simulink model "2"  (R2019a)
settings: Solver=VariableStepAuto  StartTime=0.0  StopTime=10.0  RelTol=1e-3
settings Model: Creator=TakumiShiota  LastModifiedBy=TakumiShiota

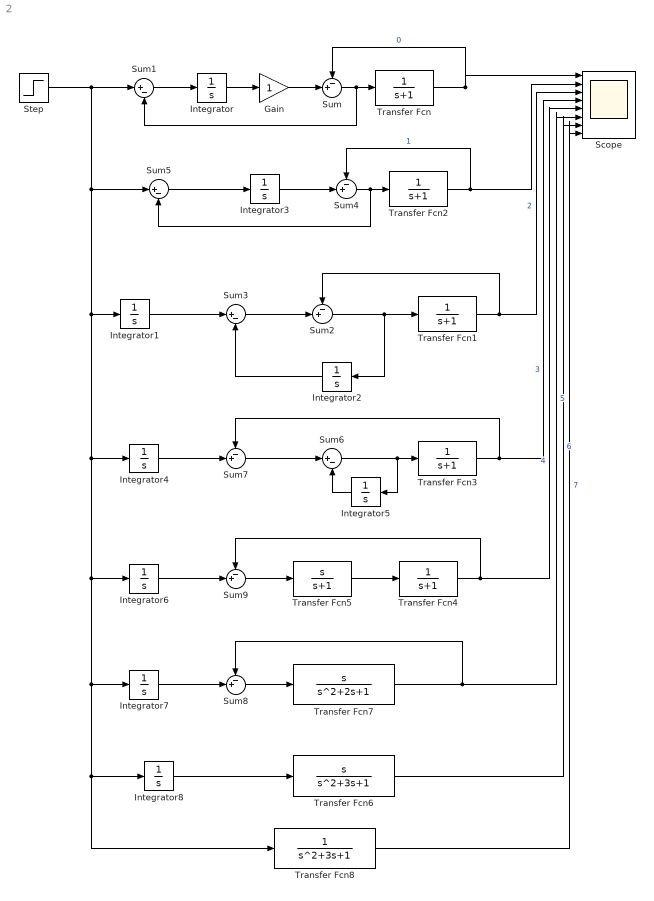
== system 2 ==
  Gain : Gain
  Integrator{,1..8} (9 alike) : Integrator
  Scope : Scope  NumInputPorts=8
  Step : Step  SampleTime=0
  Sum{,2,4,7..9} (6 alike) : Sum  Inputs=-+|
  Sum{1,3,5..6} (4 alike) : Sum  Inputs=|+-
  Transfer Fcn{,1..4} (5 alike) : TransferFcn  Denominator=[1 1]
  Transfer Fcn5 : TransferFcn  Numerator=[1 0]  Denominator=[1 1]
  Transfer Fcn6 : TransferFcn  Numerator=[1 0]  Denominator=[1 3 1]
  Transfer Fcn7 : TransferFcn  Numerator=[1 0]
  Transfer Fcn8 : TransferFcn  Denominator=[1 3 1]
  wires:
  Integrator/1 -> Gain/1
  Gain/1 -> Sum/2
  Sum/1 -> Sum1/2, Transfer Fcn/1
  Transfer Fcn/1 -> Sum/1, Scope/1  "0"
  Sum1/1 -> Integrator/1
  Sum3/1 -> Sum2/2
  Sum2/1 -> Integrator2/1, Transfer Fcn1/1
  Integrator2/1 -> Sum3/2
  Integrator1/1 -> Sum3/1
  Transfer Fcn1/1 -> Sum2/1, Scope/3  "2"
  Sum5/1 -> Integrator3/1
  Sum4/1 -> Sum5/2, Transfer Fcn2/1
  Integrator3/1 -> Sum4/2
  Transfer Fcn2/1 -> Sum4/1, Scope/2  "1"
  Integrator4/1 -> Sum7/2
  Sum6/1 -> Integrator5/1, Transfer Fcn3/1
  Transfer Fcn3/1 -> Sum7/1, Scope/4  "3"
  Sum7/1 -> Sum6/1
  Integrator5/1 -> Sum6/2
  Transfer Fcn4/1 -> Scope/5, Sum9/1  "4"
  Integrator6/1 -> Sum9/2
  Transfer Fcn5/1 -> Transfer Fcn4/1
  Sum9/1 -> Transfer Fcn5/1
  Transfer Fcn7/1 -> Scope/6, Sum8/1  "5"
  Integrator7/1 -> Sum8/2
  Sum8/1 -> Transfer Fcn7/1
  Step/1 -> Transfer Fcn8/1, Integrator8/1, Integrator7/1, Integrator6/1, Integrator4/1, Integrator1/1, Sum5/1, Sum1/1
  Transfer Fcn6/1 -> Scope/7  "6"
  Integrator8/1 -> Transfer Fcn6/1
  Transfer Fcn8/1 -> Scope/8  "7"
